simulink library "calcTangentialCoord_ul"  (R2020a)
settings: Solver=VariableStepAuto  StartTime=0.0  StopTime=10.0  RelTol=1e-3
libraries: VectorMagnitude_ul x1
settings Model: Creator=Ayaz  LastModifiedBy=Ayaz

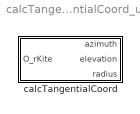
== system calcTangentialCoord_ul ==
  calcTangentialCoord : Subsystem

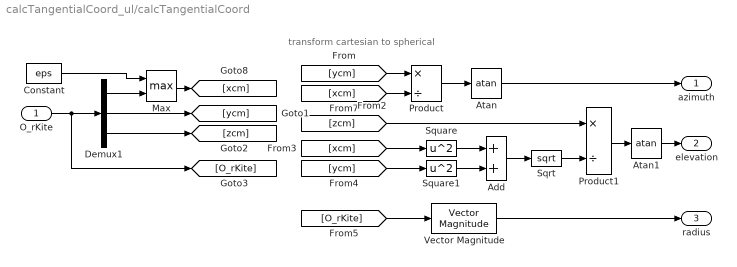
== system calcTangentialCoord_ul/calcTangentialCoord ==
  note: transform cartesian to spherical
  O_rKite : Inport
  Add : Sum
  Atan : Trigonometry  Operator=atan
  Atan1 : Trigonometry  Operator=atan
  Constant : Constant  Value=eps
  Demux1 : Demux  Outputs=3
  Max : MinMax  Function=max  Inputs=2
  Product : Product  Inputs=*/
  Product1 : Product  Inputs=*/
  Sqrt : Sqrt  SaturateOnIntegerOverflow=on
  Square : Math  Operator=square  SaturateOnIntegerOverflow=on
  Square1 : Math  Operator=square  SaturateOnIntegerOverflow=on
  Vector Magnitude : VectorMagnitude_ul/Vector Magnitude  SystemSampleTime=-1  Latency=0  AutoFrameSizeCalculation=off
  azimuth : Outport
  elevation : Outport  Port=2
  radius : Outport  Port=3
  wires:
  O_rKite/1 -> [O_rKite], Demux1/1
  Demux1/1 -> Max/2
  [ycm] -> Product/1
  [xcm] -> Product/2
  Product/1 -> Atan/1
  Atan/1 -> azimuth/1
  [xcm] -> Square/1
  [ycm] -> Square1/1
  Square1/1 -> Add/2
  Square/1 -> Add/1
  Add/1 -> Sqrt/1
  Sqrt/1 -> Product1/2
  [zcm] -> Product1/1
  Product1/1 -> Atan1/1
  [O_rKite] -> Vector Magnitude/1
  Demux1/3 -> [zcm]
  Atan1/1 -> elevation/1
  Demux1/2 -> [ycm]
  Vector Magnitude/1 -> radius/1
  Constant/1 -> Max/1
  Max/1 -> [xcm]
